simulink model "C172S_Nonlinear6Dof_V1"  (R2026a)
settings: Solver=ode4  StartTime=0  StopTime=2  FixedStep=0.01
InitFcn:
  | n6Model=c172sIntegratedNonlinearDynamicsData();
  | if ~exist('n6InitialState','var'), n6InitialState=solveC172sNonlinearTrim([],n6Model.trimModel).state; end
  | if ~exist('n6InputSignal','var'), error('n6InputSignal is required.'); end
undefined symbols (not defined in the file or in its folder): n6InitialState
settings Model: Creator=Shahi  LastModifiedBy=Shahi

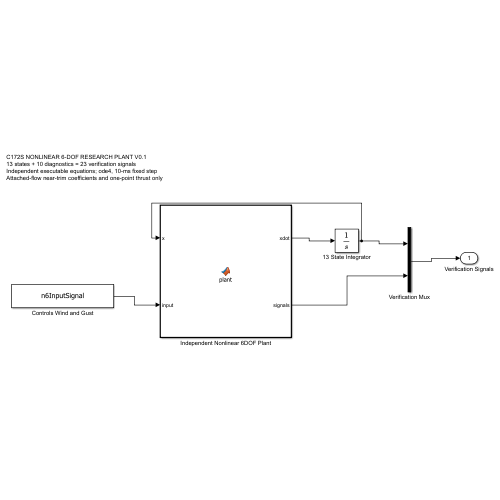
[thumbnail: Simulink's stored preview of the top-level diagram]
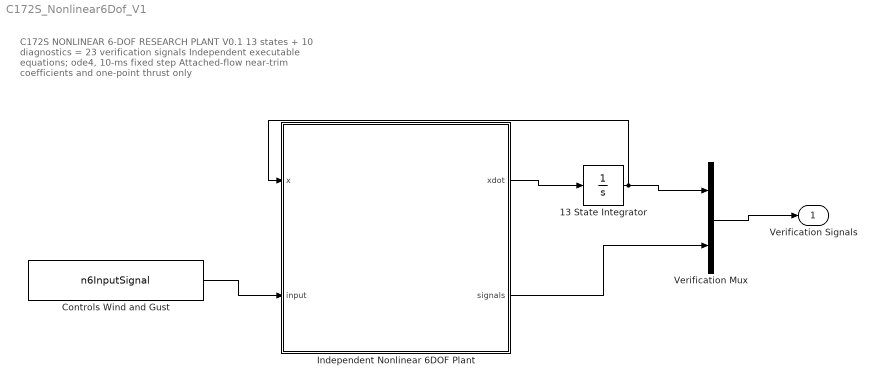
== system C172S_Nonlinear6Dof_V1 ==
  note: C172S NONLINEAR 6-DOF RESEARCH PLANT V0.1
      | 13 states + 10 diagnostics = 23 verification signals
      | Independent executable equations; ode4, 10-ms fixed step
      | Attached-flow near-trim coefficients and one-point thrust only
  13 State Integrator : Integrator  InitialCondition=n6InitialState
  Controls Wind and Gust : FromWorkspace  VariableName=n6InputSignal  Interpolate=off  OutputAfterFinalValue=Holding final value
  Independent Nonlinear 6DOF Plant : MATLAB Function  TreatAsAtomicUnit=on
  Verification Mux : Mux  Inputs=2
  Verification Signals : Outport
  wires:
  13 State Integrator/1 -> Independent Nonlinear 6DOF Plant/1(x), Verification Mux/1
  Controls Wind and Gust/1 -> Independent Nonlinear 6DOF Plant/2(input)
  Independent Nonlinear 6DOF Plant/1(xdot) -> 13 State Integrator/1
  Independent Nonlinear 6DOF Plant/2(signals) -> Verification Mux/2
  Verification Mux/1 -> Verification Signals/1

== matlab function C172S_Nonlinear6Dof_V1/Independent Nonlinear 6DOF Plant ==
  data: x input size=[13 1]; xdot output size=[13 1]; input input size=[10 1]; signals output size=[10 1]
function [xdot,signals] = plant(x,input)
%#codegen
xdot=zeros(13,1); signals=zeros(10,1);
control=input(1:4); wind=input(5:7)+input(8:10);
[f0,~,~,~,~,~,~,~,airVelocity,windBody]=evaluate(x,control,wind,0.0);
[f1,~,~,~,~,~,~,~,~,~]=evaluate(x,control,wind,1.0);
omega=x(4:6); a0=f0(1:3)+cross(omega,windBody); a1=f1(1:3)+cross(omega,windBody);
r0=alphaRate(airVelocity,a0); r1=alphaRate(airVelocity,a1); alphaDot=r0/(1-(r1-r0));
[xdot,F,M,TAS,alpha,beta,~,~,~,~]=evaluate(x,control,wind,alphaDot);
signals=[alphaDot;F;M;TAS;alpha;beta];
end
function rate=alphaRate(v,a)
rate=(v(1)*a(3)-v(3)*a(1))/(v(1)^2+v(3)^2);
end
function [xdot,F,M,TAS,alpha,beta,rho,C,airVelocity,windBody]=evaluate(x,u,wind,alphaDot)
mass=1156.6605434999999; gravity=9.8066499999999994;
I=[1424.9552348898205 0 -0;0 1828.6803192734997 0;-0 0 2956.6740184607975];
q=x(10:13); q=q/sqrt(sum(q.^2)); q0=q(1);q1=q(2);q2=q(3);q3=q(4);
C=[q0^2+q1^2-q2^2-q3^2,2*(q1*q2-q0*q3),2*(q1*q3+q0*q2);2*(q1*q2+q0*q3),q0^2-q1^2+q2^2-q3^2,2*(q2*q3-q0*q1);2*(q1*q3-q0*q2),2*(q2*q3+q0*q1),q0^2-q1^2-q2^2+q3^2];
windBody=C'*wind; airVelocity=x(1:3)-windBody; TAS=sqrt(sum(airVelocity.^2));
alpha=atan2(airVelocity(3),airVelocity(1)); beta=asin(min(1,max(-1,airVelocity(2)/TAS)));
temperature=288.14999999999998-0.0064999999999999997*(-x(9)); pressure=101325*(temperature/288.14999999999998)^(9.8066499999999994/(287.05286999999998*0.0064999999999999997)); rho=pressure/(287.05286999999998*temperature);
qbarS=0.5*rho*TAS^2*16.165128960000001; pHat=x(4)*10.91184/(2*TAS); qHat=x(5)*1.49352/(2*TAS); rHat=x(6)*10.91184/(2*TAS); adHat=alphaDot*1.49352/(2*TAS);
CL=0.40283185525292292+5.5*alpha+3.8799999999999999*qHat+1.49*adHat+0.42699999999999999*u(1);
CD=0.035628731280772659+0.25*alpha;
CY=-0.31*beta+-0.036999999999999998*pHat+0.20999999999999999*rHat+-0*u(2)+-0.187*u(3);
Cl=-0.088999999999999996*beta+-0.46999999999999997*pHat+0.096000000000000002*rHat+0.17799999999999999*u(2)+-0.0147*u(3);
Cm=-0.93794217687074832*alpha+-11.4*qHat+-4.3600000000000003*adHat+-1.26*u(1);
Cn=0.065000000000000002*beta+-0.029999999999999999*pHat+-0.099000000000000005*rHat+0.052999999999999999*u(2)+0.065699999999999995*u(3);
L=qbarS*CL;D=qbarS*CD;Y=qbarS*CY; thrust=u(4)*1543.4401413548464;
Fa=[-D*cos(alpha)+L*sin(alpha);Y;-D*sin(alpha)-L*cos(alpha)]; F=Fa+thrust*[cos(alpha);0;sin(alpha)];
M=[qbarS*10.91184*Cl;qbarS*1.49352*Cm;qbarS*10.91184*Cn];
omega=x(4:6); gravityBody=C'*[0;0;gravity]; vdot=F/mass+gravityBody-cross(omega,x(1:3));
H=I*omega; odot=I\(M-cross(omega,H)); pdot=C*x(1:3);
qv=q(2:4); Q=[-qv';q0*eye(3)+[0 -qv(3) qv(2);qv(3) 0 -qv(1);-qv(2) qv(1) 0]]; qdot=0.5*Q*omega;
xdot=[vdot;odot;pdot;qdot];
end
